simulink model "EVWITHOUTBOOSTCONVERTER"  (R2022a)
settings: Solver=ode23t  StartTime=0.0  StopTime=0.025  MaxStep=1e-3  RelTol=1e-3
undefined symbols (not defined in the file): Ion, Lithium
libraries: nesl_utility x14, fl_lib x12, sdl_lib x10, spsSeriesRLCBranchLib x5, spsDiodeLib x4, spsVoltageMeasurementLib x4, spsIGBTDiodeLib x4, simulink x3, spsMultimeterLib x3, spsPowerLib x2, spsACVoltageSourceLib x1, spsBatteryLib x1
settings Model: Creator=Arjun TM  LastModifiedBy=B SAI CHARAN TEJ
settings SolverCC: AlgebraicLoopSolver=TrustRegion
settings DataIOCC: ReturnWorkspaceOutputs=off
settings DebuggingCC: UnconnectedInputMsg=warning  UnconnectedOutputMsg=warning  UnconnectedLineMsg=warning  SFMachineParentedDataDiag=warning
settings RTWCC: DLArmComputeVersion=19.05

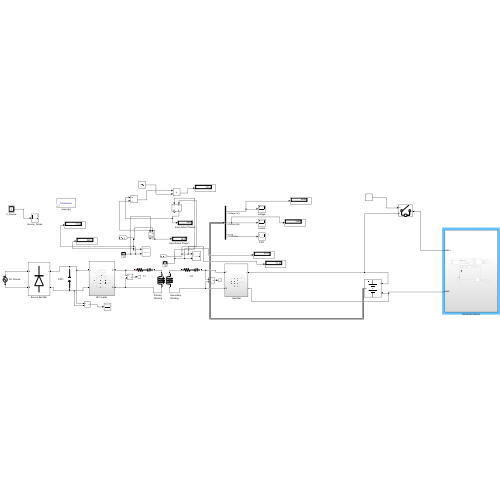
[thumbnail: Simulink's stored preview of the top-level diagram]
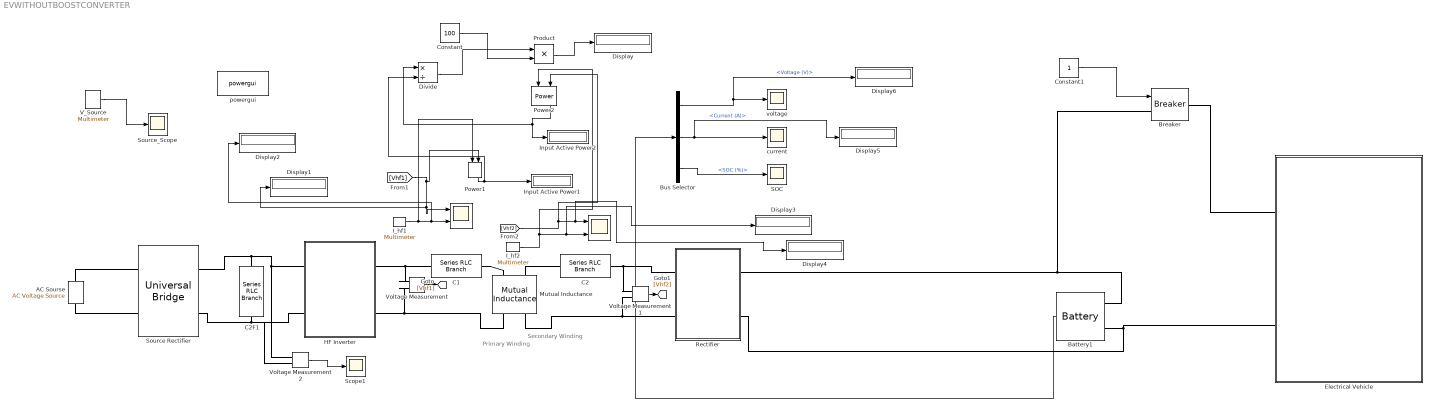
== system EVWITHOUTBOOSTCONVERTER ==
  note: Secondary
      | Winding
  note: Primary
      | Winding
  " " : Scope  NumInputPorts=2
  "   " : Scope  NumInputPorts=2
  " Rectifier" : Subsystem
  AC Sourse : spsACVoltageSourceLib/AC Voltage Source  Amplitude=230  Phase=0  Frequency=50  SampleTime=0  Measurements=Voltage  BusType=swing  Pref=10e3  Qref=0  Qmin=-inf  Qmax=+inf
  Battery1 : spsBatteryLib/Battery  BatType=Lithium-Ion  ShowTempParam=off  ThermalPreset=no  ShowAgeParam=off  NomV=72  NomQ=408.5  SOC=80  Batt_Tr=30  PresetModel=off  MaxQ=5.4  MinV=54  FullV=90.8071  Dis_rate=2.3478  R=0.13333  Normal_OP=4.8835  expZone="[85.7878     0.265304]"  current=[6.5 13 32.5]  Units=Time  Tci=20  NomT=20  T2=-30  MaxQ2=4.8  FullV2=7.1  Normal_OP2=5.655  expZone2="[6.58           1]"  Rca=0.6  ti=2000  Dp=0  Neq0=0  Tsim=1e6  Ta1=25  Qeol=5.4*0.9  Reol=0.013333*1.2  Char_age=[2.3478, 3]  Dis_age=[2.3478, 10]  N1=1500  N2=10500  N3=1000  N4=1400  Ta2=45  N5=950
  Breaker : spsBreakerLib/Breaker  InitialState=0  SwitchingTimes="[1/60  5/60]"  External=on  BreakerResistance=0.01  SnubberResistance=1e6  SnubberCapacitance=inf  Measurements=None  MoreParameters=on  NoBreakLoop=off
      settings: SourceProductBaseCode=PS
  Bus Selector : BusSelector  OutputSignals=Voltage (V),Current (A),SOC (%)
  C1 : spsSeriesRLCBranchLib/Series RLC Branch  LConnTagsString=__new0  RConnTagsString=__new0  BranchType=RC  Resistance=1e-6  Inductance=1e-3  SetiL0=off  InitialCurrent=0  Capacitance=105.74e-9  Setx0=off  InitialVoltage=0  Measurements=Branch current
  C2 : spsSeriesRLCBranchLib/Series RLC Branch  LConnTagsString=__new0  RConnTagsString=__new0  BranchType=RC  Resistance=0.001  Inductance=1e-3  SetiL0=off  InitialCurrent=0  Capacitance=109.69e-9  Setx0=off  InitialVoltage=0  Measurements=Branch current
  C2F1 : spsSeriesRLCBranchLib/Series RLC Branch  LConnTagsString=__new0  RConnTagsString=__new0  BranchType=C  Resistance=1e-6  Inductance=1e-3  SetiL0=off  InitialCurrent=0  Capacitance=500e-4  Setx0=off  InitialVoltage=0  Measurements=None
  Constant : Constant  Value=100
  Constant1 : Constant
  Display{,1..6} (7 alike) : Display
  Divide : Product  Inputs=*/
  Electrical Vehicle : Subsystem
  HF Inverter : Subsystem
  I_hf1 : spsMultimeterLib/Multimeter  L=15  sel=10  yselected={}  Gain=1  OutputType=Complex  PlotAtSimulationStop=off  PhasorSimulation=off
  I_hf2 : spsMultimeterLib/Multimeter  L=15  sel=11  yselected={}  Gain=1  OutputType=Complex  PlotAtSimulationStop=off  PhasorSimulation=off
  Input Active Power1 : Display
  Input Active Power2 : Display
  Mutual Inductance : spsMutualInductanceLib/Mutual Inductance  LConnTagsString=a|b  RConnTagsString=A|B  TypeOfMutual=Two or three windings with equal mutual terms  NumberOfWindings=3  SelfImpedance1=[1e-3 266.16e-6]  SelfImpedance2=[1e-3 256.79e-6]  ThreeWindings=off  SelfImpedance3=[ 1.1 1.1e-03]  MutualImpedance="[0  28.46e-6]"  InductanceMatrix="[1.0 0.9  0.9 ;  0.9 1.0  0.9;  0.9 0.9 1.0 ] * 1e-3"  ResistanceMatrix="[1.0 0.9  0.9 ;  0.9 1.0  0.9;  0.9 0.9 1.0 ]"  Measurements=None
      settings: SourceProductBaseCode=PS
  Power1 : spsPowerLib/Power  Freq=30000  Vinit=[1, 0]  Iinit=[1, 0]  Ts=0
      settings: SourceProductBaseCode=PS
  Power2 : spsPowerLib/Power  Freq=30000  Vinit=[1, 0]  Iinit=[1, 0]  Ts=0
      settings: SourceProductBaseCode=PS
  Product : Product
  SOC : Scope
  Scope1 : Scope
  Source Rectifier : spsUniversalBridgeLib/Universal Bridge  Arms=2  SnubberResistance=1e5  SnubberCapacitance=inf  Device=Diodes  Ron=1e-3  Lon=0  ForwardVoltages="[  0  0  ]"  ForwardVoltage=0  GTOparameters=[ 10e-6 , 20e-6 ]  IGBTparameters=[ 1e-6 , 2e-6 ]  Measurements=All voltages and currents  Measurements_2=None  converterType=Rectifier
  Source_Scope : Scope
  V_Source : spsMultimeterLib/Multimeter  L=15  sel=9  yselected={}  Gain=1  OutputType=Complex  PlotAtSimulationStop=off  PhasorSimulation=off
  Voltage Measurement : spsVoltageMeasurementLib/Voltage Measurement  PhasorSimulation=off  OutputType=Complex  PSBequivalent=0
  Voltage Measurement1 : spsVoltageMeasurementLib/Voltage Measurement  PhasorSimulation=off  OutputType=Complex  PSBequivalent=0
  Voltage Measurement2 : spsVoltageMeasurementLib/Voltage Measurement  PhasorSimulation=off  OutputType=Complex  PSBequivalent=0
  current : Scope
  powergui : spspowerguiLib/powergui  Priority=1  SimulationMode=Continuous  SampleTime=50e-5  frequency=60  Iterations=50  frequencyindice=0  Pbase=100e6  ErrMax=1e-4  UnitsV=kV  UnitsW=MW  buscounter=0  FunctionMessages=off  echomessages=off  EnableUseOfTLC=off  CurrentSourceSwitches=off  DisableSnubberDevices=off  DisableRonSwitches=off  DisableVfSwitches=off  DisplayEquations=off  AutomaticDiscreteSolvers=off  SolverType=Tustin/Backward Euler (TBE)  Interpol=off  ExternalGateDelay=off  methode=off  Ts=100  x0status=blocks  SPID=on  SwTol=0  HookPort=off  NonlinearTolerance=1e-4  nMaxIteration=100  ContinueOnMaxIteration=off  RestoreLinks=warning  ResistiveCurrentMeasurement=off  Frange=[0:2:500]  Ylog=off  Xlog=on  ShowGrid=off  save=off  variable=ZData  structure=source  ZoomFFT=off  StartTime=0.1  cycles=5  DisplayStyle=2  fundamental=50  FreqAxis=on  MaxFrequency=1000  frequencyindicesteady=1  RmsSteady=1  display=off
  voltage : Scope
  wires:
  V_Source/1 -> Source_Scope/1
  Voltage Measurement/1 -> [Vhf1]
  Voltage Measurement1/1 -> [Vhf2]
  I_hf2/1 -> Power2/2, Display3/1, "   "/2
  Bus Selector/3 -> SOC/1  "<SOC (%)>"
  Divide/1 -> Product/1
  Constant/1 -> Product/2
  Product/1 -> Display/1
  Voltage Measurement2/1 -> Scope1/1
  [Vhf1] -> Power1/1, Display1/1, " "/1
  I_hf1/1 -> Display2/1, " "/2, Power1/2
  Power1/1 -> Divide/2, Input Active Power1/1
  Battery1/1 -> Bus Selector/1
  Power2/1 -> Divide/1, Input Active Power2/1
  Bus Selector/2 -> Display5/1, current/1  "<Current (A)>"
  Constant1/1 -> Breaker/1
  [Vhf2] -> Power2/1, Display4/1, "   "/1
  Bus Selector/1 -> Display6/1, voltage/1  "<Voltage (V)>"
  connections:
  C1/RConn1 -- Mutual Inductance/LConn1
  Mutual Inductance/LConn2 -- C2/LConn1
  AC Sourse/LConn1 -- Source Rectifier/LConn2
  AC Sourse/RConn1 -- Source Rectifier/LConn1
  Source Rectifier/RConn2 -- Voltage Measurement2/LConn2 -- HF Inverter/LConn2 -- C2F1/RConn1
  C2F1/LConn1 -- Voltage Measurement2/LConn1 -- HF Inverter/LConn1 -- Source Rectifier/RConn1
  C1/LConn1 -- Voltage Measurement/LConn1 -- HF Inverter/RConn1
  Mutual Inductance/RConn1 -- Voltage Measurement/LConn2 -- HF Inverter/RConn2
  C2/RConn1 -- Voltage Measurement1/LConn1 -- " Rectifier"/LConn1
  Mutual Inductance/RConn2 -- Voltage Measurement1/LConn2 -- " Rectifier"/LConn2
  " Rectifier"/RConn2 -- Electrical Vehicle/LConn2 -- Battery1/LConn2
  Electrical Vehicle/LConn1 -- Breaker/RConn1
  " Rectifier"/RConn1 -- Breaker/LConn1 -- Battery1/LConn1

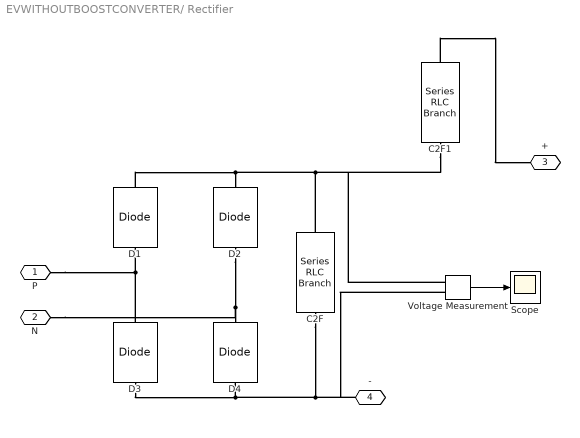
== system EVWITHOUTBOOSTCONVERTER/ Rectifier ==
  C2F : spsSeriesRLCBranchLib/Series RLC Branch  LConnTagsString=__new0  RConnTagsString=__new0  BranchType=C  Resistance=1e-6  Inductance=1e-3  SetiL0=off  InitialCurrent=0  Capacitance=300e-6  Setx0=off  InitialVoltage=0  Measurements=Branch voltage
  C2F1 : spsSeriesRLCBranchLib/Series RLC Branch  LConnTagsString=__new0  RConnTagsString=__new0  BranchType=R  Resistance=1e-6  Inductance=1e-3  SetiL0=off  InitialCurrent=0  Capacitance=300e-6  Setx0=off  InitialVoltage=0  Measurements=Branch voltage
  D{1..4} (4 alike) : spsDiodeLib/Diode  Ron=0.001  Lon=0  Vf=0.8  IC=0  UseSnubber=0  Rs=500  Cs=250e-9  Measurements=off
  Scope : Scope
  Voltage Measurement : spsVoltageMeasurementLib/Voltage Measurement  PhasorSimulation=off  OutputType=Complex  PSBequivalent=0
  P : PMIOPort  Side=Left
  N : PMIOPort  Port=2  Side=Left
  + : PMIOPort  Port=3  Side=Right
  - : PMIOPort  Port=4  Side=Right
  wires:
  Voltage Measurement/1 -> Scope/1
  connections:
  D1/RConn1 -- C2F1/RConn1 -- Voltage Measurement/LConn1 -- C2F/LConn1 -- D2/RConn1
  D3/RConn1 -- P/RConn1 -- D1/LConn1
  C2F/RConn1 -- Voltage Measurement/LConn2 -- -/RConn1 -- D3/LConn1 -- D4/LConn1
  D2/LConn1 -- N/RConn1 -- D4/RConn1
  C2F1/LConn1 -- +/RConn1

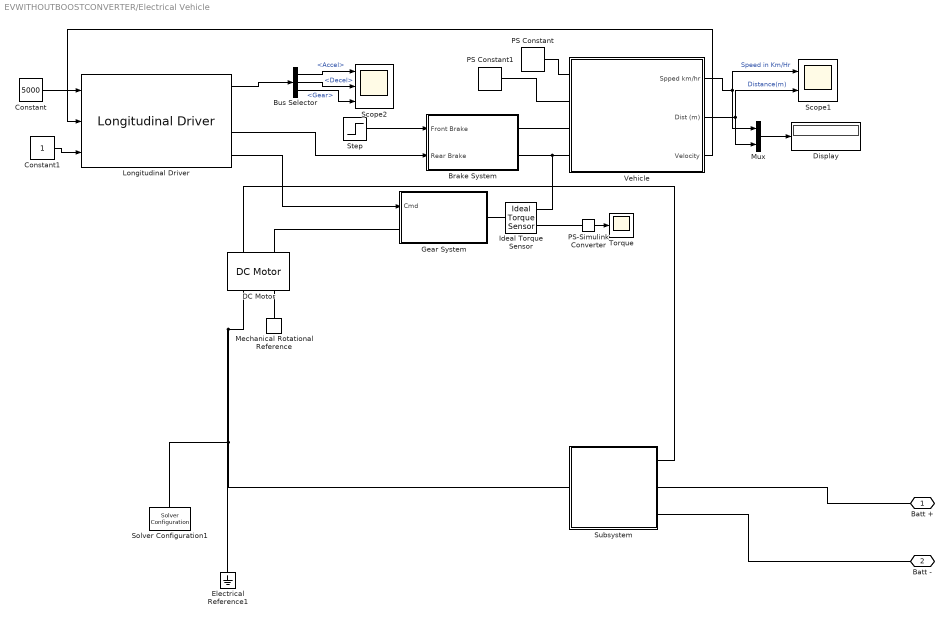
== system EVWITHOUTBOOSTCONVERTER/Electrical Vehicle ==
  Brake System : Subsystem
  Bus Selector : BusSelector  OutputSignals=Accel,Decel,Gear
  Constant : Constant  Value=5000
  Constant1 : Constant
  DC Motor : ee_lib/Electromechanical/Brushed Motors/DC Motor  field_option=ee.enum.field_option.pm  Rf=100 Ohm  Lf=1 H  Laf=0.15 H  If0=0 A  parameterization=ee.enum.dcparam_option.load_speed  Ra=3.9 Ohm  La=0.005 H  emf_or_torque=ee.enum.emf_or_torque.kv  Kv=0.072e-3 V/rpm  Ki=6.876e-4 N*m/A  T_stall=0.24e-3 N*m  w_max=9000 rpm  w_rated=8000 rpm  P_rated=5 kW  V_rated=72 V  lam_param=ee.enum.lam_param.damping  i_noload=0 A  V_i_noload=1.5 V  J=0.01 g*cm^2  lam=0 N*m/(rad/s)  speed0=0 rpm  enable_fault_armature=simscape.enum.onoff.off  rev_faulted=1 / 3  G_faulted_armature=1e-5 S  fault_trigger_armature=ee.enum.faults.faultTrigger.temporal  t_fault_armature=1 s  max_permissible_current_armature=inf A  t_fail_on_current_armature=1 s  enable_fault_field=simscape.enum.onoff.off  G_faulted_field=1e-5 S  fault_trigger_field=ee.enum.faults.faultTrigger.temporal  t_fault_field=1 s  max_permissible_current_field=inf A  t_fail_on_current_field=1 s  fault_action=simscape.enum.assert.action.none  alpha=3.93e-3 1/K  Tmeas=25 degC  thermal_mass=100 J/K  initial_temperature=25 degC
  Display : Display
  Electrical Reference1 : fl_lib/Electrical/Electrical Elements/Electrical Reference
  Gear System : Subsystem
  Ideal Torque Sensor : fl_lib/Mechanical/Mechanical Sensors/Ideal Torque Sensor
  Longitudinal Driver : autolibshared/Longitudinal Driver  extAccelOvr=off  extDecelOvr=off  extAccelHld=off  extDecelHld=off  extAccelZero=off  extDecelZero=off  cntrlType=PI  shftType=None  velUnits=m/s  gearOut=on  Kp=15  Ki=1  Kff=.05  Kg=.01  VehVelVec=[0 100]  KffVec=[.1 .1]  KpVec=[10 10]  KiVec=[5 5]  KgVec=[0 0]  m=1500  Kpt=3000  tau=.1  L=2  aR=200  bR=2.5  cR=.5  g=9.81  vnom=100  Kaw=.1  tauerr=.03  tauPt=2  GearInit=0  tShift=.1  pdlVec=[0.1 0.4 0.5 0.9]  upShftTbl=[-1 12.9375 26.4375 39.9375 51.18749999999999 62.4375 72.84375 83.25;-1 16.3125 29.8125 43.3125 54.5624 65.8125 76.78125 87.75;-1 19.6875 33.1875 46.68749999999999 57.9375 69.1875 80.71875 92.25;-1 33 52.5 77.25 100.5 138.75 161.875 185]  dwnShftTbl=[1 9.5625 23.0625 36.5625 47.8125 59.0625 68.90625 78.75;1 12.9375 26.4375 39.9375 51.18749999999999 62.4375 72.84375 83.25;1 16.3125 29.8125 43.3125 54.562499 65.8125 76.78125 87.75;1 19.6875 33.1875 46.68749999999999 57.9375 69.1875 80.71875 92.25]  tClutch=.5  tRev=.5  tPark=120  aMode=1  UpGearVec="[0  1  2  3  4  5  6  7]"  DownGearVec="[1  2  3  4  5  6  7  8]"
      settings: SourceProductBaseCode=PW,DR,MT,UV,VE
  Mechanical Rotational Reference : fl_lib/Mechanical/Rotational Elements/Mechanical Rotational Reference
  Mux : Mux  Inputs=2
  PS Constant : fl_lib/Physical Signals/Sources/PS Constant  constant=0
  PS Constant1 : fl_lib/Physical Signals/Sources/PS Constant  constant=0
  PS-Simulink Converter : nesl_utility/PS-Simulink Converter  PhysicalDomain=network_engine_domain  SubClassName=ps_output  LeftPortType=input  RightPortType=output  PseudoPeriodic=off  Frequencies=[]  VectorFormat=1-D array  Unit=inherit  AffineConversion=off
      settings: SourceProductBaseCode=PW,SS
  Scope1 : Scope  NumInputPorts=2
  Scope2 : Scope  NumInputPorts=3
  Solver Configuration1 : nesl_utility/Solver Configuration  PhysicalDomain=network_engine_domain  SubClassName=solver  LeftPortType=input  RightPortType=generic  Tones=[]  Harmonics=[]  SimulateNoise=off  Profile=off  UseLocalSampling=off  EnableSwitchedLinearOptims=on  FrequencyDomain=off  UseCCode=off  RelTol=0.001  AbsTol=1e-06  MinStep=1e-09  ToWorkspace=off  RevertToSquareIcSolve=off  NumHomotopyIterations=100  PhasorMode=off  PhasorModeNumHarmonics=1  IndexReductionMethod=DerivativeReplacement  DoDC=off  ResidualTolerance=1e-09  UseLocalSolver=off  LocalSolverChoice=NE_BACKWARD_EULER_ADVANCER  LocalSolverSampleTime=1e-7  DoFixedCost=on  MaxNonlinIter=3  MaxModeIter=2  ComputeImpulses=off  ImpulseIterations=2  LinearAlgebra=Sparse  LinearAlgebraNumThread=0  EquationFormulation=NE_TIME_EF  DelaysMemoryBudget=1024  AutomaticFiltering=on  FilteringTimeConstant=0.001  PartitionStorageMethod=AS_NEEDED  PartitionMemoryBudget=1024  PartitionMethod=FAST
      settings: SourceProductBaseCode=PW,SS
  Step : Step  Time=75  After=100  SampleTime=0
  Subsystem : Subsystem
  Torque : Scope
  Vehicle : Subsystem
  Batt + : PMIOPort  Side=Left
  Batt - : PMIOPort  Port=2  Side=Left
  wires:
  Step/1 -> Brake System/1(Front Brake)
  Bus Selector/2 -> Scope2/2  "<Decel>"
  Constant1/1 -> Longitudinal Driver/3
  Vehicle/2(Dist (m)) -> Mux/2, Scope1/2  "Distance(m)"
  PS-Simulink Converter/1 -> Torque/1
  Vehicle/1(Spped km/hr) -> Scope1/1, Mux/1  "Speed in Km/Hr"
  Bus Selector/1 -> Scope2/1  "<Accel>"
  Constant/1 -> Longitudinal Driver/1
  Longitudinal Driver/1 -> Bus Selector/1
  Mux/1 -> Display/1
  Vehicle/3(Velocity) -> Longitudinal Driver/2
  Longitudinal Driver/3 -> Brake System/2(Rear Brake)
  Longitudinal Driver/4 -> Gear System/1(Cmd)
  Bus Selector/3 -> Scope2/3  "<Gear>"
  connections:
  Solver Configuration1/RConn1 -- Electrical Reference1/LConn1 -- DC Motor/RConn1 -- Subsystem/LConn1
  PS Constant/RConn1 -- Vehicle/LConn1
  Brake System/RConn2 -- Ideal Torque Sensor/RConn1 -- Vehicle/LConn4
  PS Constant1/RConn1 -- Vehicle/LConn2
  Ideal Torque Sensor/RConn2 -- PS-Simulink Converter/LConn1
  Gear System/RConn1 -- Ideal Torque Sensor/LConn1
  Brake System/RConn1 -- Vehicle/LConn3
  Mechanical Rotational Reference/LConn1 -- DC Motor/RConn2
  Batt +/RConn1 -- Subsystem/RConn2
  Batt -/RConn1 -- Subsystem/RConn3
  Gear System/LConn1 -- DC Motor/LConn2
  DC Motor/LConn1 -- Subsystem/RConn1

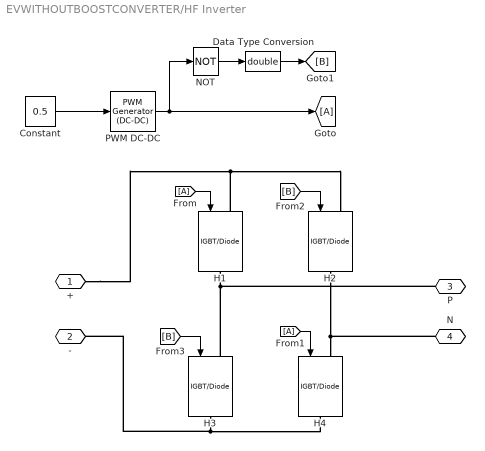
== system EVWITHOUTBOOSTCONVERTER/HF Inverter ==
  Constant : Constant  Value=0.5
  Data Type Conversion : DataTypeConversion  OutDataTypeStr=double  SaturateOnIntegerOverflow=off  RndMeth=Floor
  From : From
  From1 : From
  Goto : Goto
  H{1..4} (4 alike) : spsIGBTDiodeLib/IGBT//Diode  Ron=1e-3  Rs=1e5  Cs=inf  Measurements=off
  "NOT " : Logic  Operator=NOT  IconShape=distinctive  AllPortsSameDT=off  OutDataTypeStr=boolean
  PWM DC-DC : spsPWMGeneratorDCDCLib/PWM Generator (DC-DC)  Fsw=30000  Ts=0
  + : PMIOPort  Side=Left
  - : PMIOPort  Port=2  Side=Left
  P : PMIOPort  Port=3  Side=Right
  N : PMIOPort  Port=4  Side=Right
  wires:
  [B] -> H2/1
  [B] -> H3/1
  From1/1 -> H4/1
  From/1 -> H1/1
  "NOT "/1 -> Data Type Conversion/1
  Constant/1 -> PWM DC-DC/1
  Data Type Conversion/1 -> [B]
  PWM DC-DC/1 -> "NOT "/1, Goto/1
  connections:
  H1/LConn1 -- H2/LConn1 -- +/RConn1
  H2/RConn1 -- N/RConn1 -- H4/LConn1
  H3/RConn1 -- -/RConn1 -- H4/RConn1
  H3/LConn1 -- P/RConn1 -- H1/RConn1

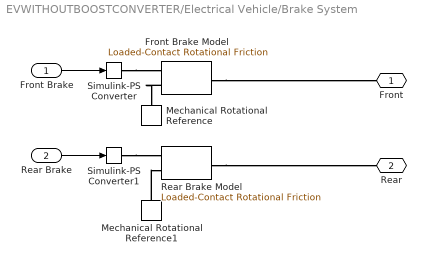
== system EVWITHOUTBOOSTCONVERTER/Electrical Vehicle/Brake System ==
  Front Brake : Inport
  Rear Brake : Inport  Port=2
  Front Brake Model : sdl_lib/Brakes & Detents/Rotational/Loaded-Contact Rotational Friction  geometry_model=sdl.enum.friction_geometry.radius  r_eff=280 mm  d_o=150 mm  d_i=100 mm  friction_model=sdl.enum.friction_model_TLU_thermal.fixed  mu_w_vector=[0, 100, 1000] rad/s  temperature_TLU=[280, 300, 320] K  mu_static=0.35  mu_static_vector=[.4, .38, .36]  mu_coulomb=0.3  mu_coulomb_vector=[.3, .22, .19]  mu_coulomb_temp_vector=[.3, .28, .25]  mu_coulomb_matrix=[.34, .32, .3; .3, .28, .25; .25, .2, .15]  mu_interp_method=simscape.enum.interpolation.linear  mu_extrap_method=simscape.enum.extrapolation.linear  w_tol=0.001 rad/s  force_min=1 N  mu_visc=0 N*m/(rad/s)  initial_state_locked=sdl.enum.initial_lock.unlocked  enable_faults=simscape.enum.onoff.off  fault_type=sdl.enum.clutchFault.lock  external_fault=simscape.enum.onoff.off  temporal_fault=simscape.enum.onoff.off  fault_time=5 s  report_fault=simscape.enum.assert.action.none  thermal_mass=50 kJ/K  T_init=300 K
      settings: SourceProductBaseCode=LD  InternalSimscapePortConfiguration="{\"Bottom\":[],\"Left\":[{\"id\":\"N\",\"label\":\"N\",\"type\":\"input\"},{\"id\":\"B\",\"label\":\"B\",\"type\":\"foundation.mechanical.rotational.rotational\"}],\"Right\":[{\"id\":\"F\",\"label\":\"F\",\"type\":\"foundation.mechanical.rotational.rotational\"}],\"Top\":[]}"
  Mechanical Rotational Reference : fl_lib/Mechanical/Rotational Elements/Mechanical Rotational Reference
  Mechanical Rotational Reference1 : fl_lib/Mechanical/Rotational Elements/Mechanical Rotational Reference
  Rear Brake Model : sdl_lib/Brakes & Detents/Rotational/Loaded-Contact Rotational Friction  geometry_model=sdl.enum.friction_geometry.radius  r_eff=280 mm  d_o=150 mm  d_i=100 mm  friction_model=sdl.enum.friction_model_TLU_thermal.fixed  mu_w_vector=[0, 100, 1000] rad/s  temperature_TLU=[280, 300, 320] K  mu_static=0.35  mu_static_vector=[.4, .38, .36]  mu_coulomb=0.3  mu_coulomb_vector=[.3, .22, .19]  mu_coulomb_temp_vector=[.3, .28, .25]  mu_coulomb_matrix=[.34, .32, .3; .3, .28, .25; .25, .2, .15]  mu_interp_method=simscape.enum.interpolation.linear  mu_extrap_method=simscape.enum.extrapolation.linear  w_tol=0.001 rad/s  force_min=1 N  mu_visc=0 N*m/(rad/s)  initial_state_locked=sdl.enum.initial_lock.unlocked  enable_faults=simscape.enum.onoff.off  fault_type=sdl.enum.clutchFault.lock  external_fault=simscape.enum.onoff.off  temporal_fault=simscape.enum.onoff.off  fault_time=5 s  report_fault=simscape.enum.assert.action.none  thermal_mass=50 kJ/K  T_init=300 K
      settings: SourceProductBaseCode=LD  InternalSimscapePortConfiguration="{\"Bottom\":[],\"Left\":[{\"id\":\"N\",\"label\":\"N\",\"type\":\"input\"},{\"id\":\"B\",\"label\":\"B\",\"type\":\"foundation.mechanical.rotational.rotational\"}],\"Right\":[{\"id\":\"F\",\"label\":\"F\",\"type\":\"foundation.mechanical.rotational.rotational\"}],\"Top\":[]}"
  Simulink-PS Converter : nesl_utility/Simulink-PS Converter  PhysicalDomain=network_engine_domain  SubClassName=ps_input  LeftPortType=input  RightPortType=output  PseudoPeriodic=off  Frequencies=[]  NoiseDistribution=none  NoiseParameters=[]  Unit=1  AffineConversion=off  FilteringAndDerivatives=provide  SimscapeFilterOrder=1  InputFilterTimeConstant=0.001  UdotUserProvided=0
      settings: SourceProductBaseCode=PW,SS
  Simulink-PS Converter1 : nesl_utility/Simulink-PS Converter  PhysicalDomain=network_engine_domain  SubClassName=ps_input  LeftPortType=input  RightPortType=output  PseudoPeriodic=off  Frequencies=[]  NoiseDistribution=none  NoiseParameters=[]  Unit=1  AffineConversion=off  FilteringAndDerivatives=provide  SimscapeFilterOrder=1  InputFilterTimeConstant=0.001  UdotUserProvided=0
      settings: SourceProductBaseCode=PW,SS
  Front : PMIOPort  Side=Right
  Rear : PMIOPort  Port=2  Side=Right
  wires:
  Rear Brake/1 -> Simulink-PS Converter1/1
  Front Brake/1 -> Simulink-PS Converter/1
  connections:
  Simulink-PS Converter1/RConn1 -- Rear Brake Model/LConn1
  Mechanical Rotational Reference1/LConn1 -- Rear Brake Model/LConn2
  Rear Brake Model/RConn1 -- Rear/RConn1
  Front Brake Model/LConn2 -- Mechanical Rotational Reference/LConn1
  Simulink-PS Converter/RConn1 -- Front Brake Model/LConn1
  Front Brake Model/RConn1 -- Front/RConn1

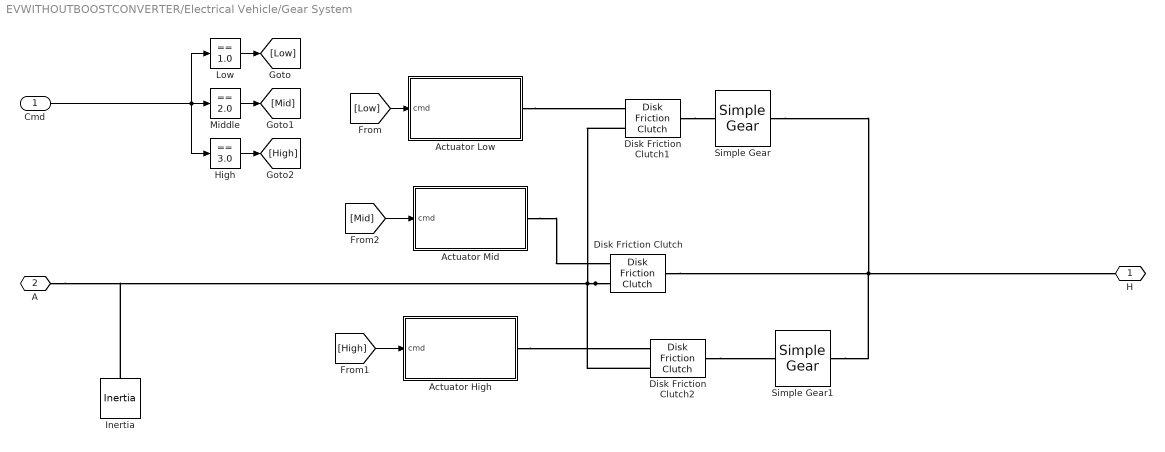
== system EVWITHOUTBOOSTCONVERTER/Electrical Vehicle/Gear System ==
  Cmd : Inport
  Actuator High : Subsystem
  Actuator Low : Subsystem
  Actuator Mid : Subsystem
  Disk Friction Clutch : sdl_lib/Clutches/Disk Friction Clutch  geometry_model=sdl.enum.friction_geometry.radius  r_eff=130 mm  d_o=150 mm  d_i=100 mm  nS=4  piston_area=0.001 m^2  unidirectional=sdl.enum.directionality.bidirectional  friction_model=sdl.enum.friction_model_TLU_thermal.fixed  mu_w_vector=[0, 100, 1000] rad/s  temperature_TLU=[280, 300, 320] K  mu_static=0.35  mu_static_vector=[.4, .38, .36]  mu_coulomb=0.3  mu_coulomb_vector=[.3, .22, .19]  mu_coulomb_temp_vector=[.3, .28, .25]  mu_coulomb_matrix=[.34, .32, .3; .3, .28, .25; .25, .2, .15]  mu_interp_method=simscape.enum.interpolation.linear  mu_extrap_method=simscape.enum.extrapolation.linear  d_f=1  w_tol=0.001 rad/s  pressure_min=100 Pa  mu_visc=0 N*m/(rad/s)  initial_state_locked=sdl.enum.initial_lock.unlocked  enable_faults=simscape.enum.onoff.off  fault_type=sdl.enum.clutchFault.lock  external_fault=simscape.enum.onoff.off  temporal_fault=simscape.enum.onoff.off  fault_time=5 s  report_fault=simscape.enum.assert.action.none  thermal_mass=50 kJ/K  T_init=300 K
      settings: SourceProductBaseCode=LD  InternalSimscapePortConfiguration="{\"Bottom\":[],\"Left\":[{\"id\":\"P\",\"label\":\"P\",\"type\":\"input\"},{\"id\":\"B\",\"label\":\"B\",\"type\":\"foundation.mechanical.rotational.rotational\"}],\"Right\":[{\"id\":\"F\",\"label\":\"F\",\"type\":\"foundation.mechanical.rotational.rotational\"}],\"Top\":[]}"
  Disk Friction Clutch1 : sdl_lib/Clutches/Disk Friction Clutch  geometry_model=sdl.enum.friction_geometry.radius  r_eff=130 mm  d_o=150 mm  d_i=100 mm  nS=4  piston_area=0.001 m^2  unidirectional=sdl.enum.directionality.bidirectional  friction_model=sdl.enum.friction_model_TLU_thermal.fixed  mu_w_vector=[0, 100, 1000] rad/s  temperature_TLU=[280, 300, 320] K  mu_static=0.35  mu_static_vector=[.4, .38, .36]  mu_coulomb=0.3  mu_coulomb_vector=[.3, .22, .19]  mu_coulomb_temp_vector=[.3, .28, .25]  mu_coulomb_matrix=[.34, .32, .3; .3, .28, .25; .25, .2, .15]  mu_interp_method=simscape.enum.interpolation.linear  mu_extrap_method=simscape.enum.extrapolation.linear  d_f=1  w_tol=0.001 rad/s  pressure_min=100 Pa  mu_visc=0 N*m/(rad/s)  initial_state_locked=sdl.enum.initial_lock.unlocked  enable_faults=simscape.enum.onoff.off  fault_type=sdl.enum.clutchFault.lock  external_fault=simscape.enum.onoff.off  temporal_fault=simscape.enum.onoff.off  fault_time=5 s  report_fault=simscape.enum.assert.action.none  thermal_mass=50 kJ/K  T_init=300 K
      settings: SourceProductBaseCode=LD  InternalSimscapePortConfiguration="{\"Bottom\":[],\"Left\":[{\"id\":\"P\",\"label\":\"P\",\"type\":\"input\"},{\"id\":\"B\",\"label\":\"B\",\"type\":\"foundation.mechanical.rotational.rotational\"}],\"Right\":[{\"id\":\"F\",\"label\":\"F\",\"type\":\"foundation.mechanical.rotational.rotational\"}],\"Top\":[]}"
  Disk Friction Clutch2 : sdl_lib/Clutches/Disk Friction Clutch  geometry_model=sdl.enum.friction_geometry.radius  r_eff=130 mm  d_o=150 mm  d_i=100 mm  nS=4  piston_area=0.001 m^2  unidirectional=sdl.enum.directionality.bidirectional  friction_model=sdl.enum.friction_model_TLU_thermal.fixed  mu_w_vector=[0, 100, 1000] rad/s  temperature_TLU=[280, 300, 320] K  mu_static=0.35  mu_static_vector=[.4, .38, .36]  mu_coulomb=0.3  mu_coulomb_vector=[.3, .22, .19]  mu_coulomb_temp_vector=[.3, .28, .25]  mu_coulomb_matrix=[.34, .32, .3; .3, .28, .25; .25, .2, .15]  mu_interp_method=simscape.enum.interpolation.linear  mu_extrap_method=simscape.enum.extrapolation.linear  d_f=1  w_tol=0.001 rad/s  pressure_min=100 Pa  mu_visc=0 N*m/(rad/s)  initial_state_locked=sdl.enum.initial_lock.unlocked  enable_faults=simscape.enum.onoff.off  fault_type=sdl.enum.clutchFault.lock  external_fault=simscape.enum.onoff.off  temporal_fault=simscape.enum.onoff.off  fault_time=5 s  report_fault=simscape.enum.assert.action.none  thermal_mass=50 kJ/K  T_init=300 K
      settings: SourceProductBaseCode=LD  InternalSimscapePortConfiguration="{\"Bottom\":[],\"Left\":[{\"id\":\"P\",\"label\":\"P\",\"type\":\"input\"},{\"id\":\"B\",\"label\":\"B\",\"type\":\"foundation.mechanical.rotational.rotational\"}],\"Right\":[{\"id\":\"F\",\"label\":\"F\",\"type\":\"foundation.mechanical.rotational.rotational\"}],\"Top\":[]}"
  High : simulink/Logic and Bit Operations/Compare To Constant  relop===  const=3.0  OutDataTypeStr=boolean
  Inertia : fl_lib/Mechanical/Rotational Elements/Inertia  inertia=0.01 kg*m^2  num_ports=foundation.enum.numPorts2.one  w_specify=off  w_priority=High  w=0 rad/s  w_nominal_specify=off  w_nominal_unit=rad/s  w_nominal_value=1  t_specify=off  t_priority=None  t=0 N*m  t_nominal_specify=off  t_nominal_unit=N*m  t_nominal_value=1
  Low : simulink/Logic and Bit Operations/Compare To Constant  relop===  const=1.0  OutDataTypeStr=boolean
  Middle : simulink/Logic and Bit Operations/Compare To Constant  relop===  const=2.0  OutDataTypeStr=boolean
  Simple Gear : sdl_lib/Gears/Simple Gear  ratio=3/2  rotation_direction=3-2*(1)  friction_model=sdl.enum.gear_efficiencies_load.off  T_noload=0.1 N*m  T_nom=5 N*m  efficiency_nom=0.8  efficiency=0.8  temperature_TLU=[280, 300, 320] K  load_TLU=[1, 5, 10] N*m  efficiency_TLU=[.95, .9, .85]  efficiency_TLU2=[.85, .8, .75; .95, .9, .85; .85, .8, .7]  w_thr=0.01 rad/s  pwr_thr=0.001 W  backlash_model=sdl.enum.backlashModel.Off  backlash_distance=1e-3 mm  x0=0 mm  r_base=0.1 m  hardstop_model=simscape.enum.hardstop.smooth  transition=1e-4 mm  backlash_stiffness=1e7 N/m  backlash_damping=1e6 N*s/m  e=0  v_tol=0.001 m/s  mu_visc=[0, 0] N*m/(rad/s)  enable_faults=simscape.enum.onoff.off  efficiency_fault=0.05  external_fault=simscape.enum.onoff.off  temporal_fault=simscape.enum.onoff.off  fault_time=5 s  fault_angles=pi / 12 rad  report_fault=(1)-1  thermal_mass=50 J/K  temperature_specify=off  temperature_priority=High  temperature=300 K  temperature_nominal_specify=off  temperature_nominal_unit=K  temperature_nominal_value=1  x_backlash_specify=off  x_backlash_priority=None  x_backlash=0 mm  x_backlash_nominal_specify=off  x_backlash_nominal_unit=mm  x_backlash_nominal_value=1  f_hardstop_specify=off  f_hardstop_priority=None  f_hardstop=0 N  f_hardstop_nominal_specify=off  f_hardstop_nominal_unit=N  f_hardstop_nominal_value=1  v_backlash_specify=off  v_backlash_priority=None  v_backlash=0 m/s  v_backlash_nominal_specify=off  v_backlash_nominal_unit=m/s  v_backlash_nominal_value=1
  Simple Gear1 : sdl_lib/Gears/Simple Gear  ratio=2/3  rotation_direction=3-2*(1)  friction_model=sdl.enum.gear_efficiencies_load.off  T_noload=0.1 N*m  T_nom=5 N*m  efficiency_nom=0.8  efficiency=0.8  temperature_TLU=[280, 300, 320] K  load_TLU=[1, 5, 10] N*m  efficiency_TLU=[.95, .9, .85]  efficiency_TLU2=[.85, .8, .75; .95, .9, .85; .85, .8, .7]  w_thr=0.01 rad/s  pwr_thr=0.001 W  backlash_model=sdl.enum.backlashModel.Off  backlash_distance=1e-3 mm  x0=0 mm  r_base=0.1 m  hardstop_model=simscape.enum.hardstop.smooth  transition=1e-4 mm  backlash_stiffness=1e7 N/m  backlash_damping=1e6 N*s/m  e=0  v_tol=0.001 m/s  mu_visc=[0, 0] N*m/(rad/s)  enable_faults=simscape.enum.onoff.off  efficiency_fault=0.05  external_fault=simscape.enum.onoff.off  temporal_fault=simscape.enum.onoff.off  fault_time=5 s  fault_angles=pi / 12 rad  report_fault=(1)-1  thermal_mass=50 J/K  temperature_specify=off  temperature_priority=High  temperature=300 K  temperature_nominal_specify=off  temperature_nominal_unit=K  temperature_nominal_value=1  x_backlash_specify=off  x_backlash_priority=None  x_backlash=0 mm  x_backlash_nominal_specify=off  x_backlash_nominal_unit=mm  x_backlash_nominal_value=1  f_hardstop_specify=off  f_hardstop_priority=None  f_hardstop=0 N  f_hardstop_nominal_specify=off  f_hardstop_nominal_unit=N  f_hardstop_nominal_value=1  v_backlash_specify=off  v_backlash_priority=None  v_backlash=0 m/s  v_backlash_nominal_specify=off  v_backlash_nominal_unit=m/s  v_backlash_nominal_value=1
  H : PMIOPort  Side=Right
  A : PMIOPort  Port=2  Side=Left
  wires:
  [High] -> Actuator High/1(cmd)
  Cmd/1 -> High/1, Middle/1, Low/1
  Middle/1 -> [Mid]
  Low/1 -> [Low]
  [Low] -> Actuator Low/1(cmd)
  High/1 -> [High]
  [Mid] -> Actuator Mid/1(cmd)
  connections:
  Actuator High/RConn1 -- Disk Friction Clutch2/LConn1
  Actuator Mid/RConn1 -- Disk Friction Clutch/LConn1
  Disk Friction Clutch/LConn2 -- Inertia/LConn1 -- A/RConn1 -- Disk Friction Clutch2/LConn2 -- Disk Friction Clutch1/LConn2
  Actuator Low/RConn1 -- Disk Friction Clutch1/LConn1
  Disk Friction Clutch/RConn1 -- H/RConn1 -- Simple Gear/RConn1 -- Simple Gear1/RConn1
  Disk Friction Clutch1/RConn1 -- Simple Gear/LConn1
  Disk Friction Clutch2/RConn1 -- Simple Gear1/LConn1

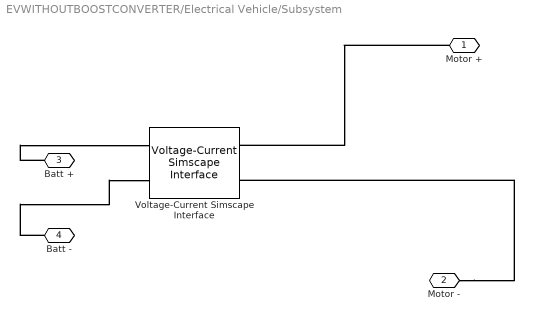
== system EVWITHOUTBOOSTCONVERTER/Electrical Vehicle/Subsystem ==
  Voltage-Current Simscape Interface : spsVoltageCurrentSimscapeInterfaceLib/Voltage-Current Simscape Interface  DFT=off  Fmode=First-order input filtering  T=1e-6  Ts=50e-6  i0=0  v0=0  Sd=Specialized Power Systems side  Measurements=off
      settings: SourceProductBaseCode=PS
  Motor + : PMIOPort  Side=Right
  Motor - : PMIOPort  Port=2  Side=Left
  Batt + : PMIOPort  Port=3  Side=Right
  Batt - : PMIOPort  Port=4  Side=Right
  connections:
  Motor -/RConn1 -- Voltage-Current Simscape Interface/RConn2
  Batt +/RConn1 -- Voltage-Current Simscape Interface/LConn1
  Batt -/RConn1 -- Voltage-Current Simscape Interface/LConn2
  Motor +/RConn1 -- Voltage-Current Simscape Interface/RConn1

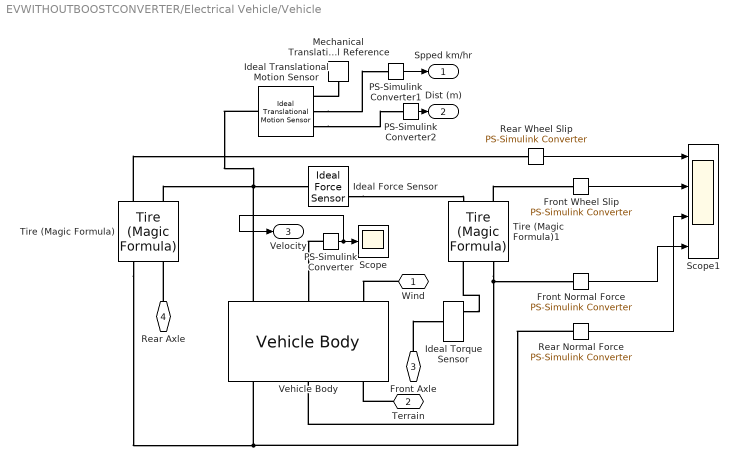
== system EVWITHOUTBOOSTCONVERTER/Electrical Vehicle/Vehicle ==
  Front Normal Force : nesl_utility/PS-Simulink Converter  PhysicalDomain=network_engine_domain  SubClassName=ps_output  LeftPortType=input  RightPortType=output  PseudoPeriodic=off  Frequencies=[]  VectorFormat=1-D array  Unit=N  AffineConversion=off
      settings: SourceProductBaseCode=PW,SS
  Front Wheel Slip : nesl_utility/PS-Simulink Converter  PhysicalDomain=network_engine_domain  SubClassName=ps_output  LeftPortType=input  RightPortType=output  PseudoPeriodic=off  Frequencies=[]  VectorFormat=1-D array  Unit=m  AffineConversion=off
      settings: SourceProductBaseCode=PW,SS
  Ideal Force Sensor : fl_lib/Mechanical/Mechanical Sensors/Ideal Force Sensor
  Ideal Torque Sensor : fl_lib/Mechanical/Mechanical Sensors/Ideal Torque Sensor
  Ideal Translational Motion Sensor : fl_lib/Mechanical/Mechanical Sensors/Ideal Translational Motion Sensor  offset=0 m
  Mechanical Translational Reference : fl_lib/Mechanical/Translational Elements/Mechanical Translational Reference
  PS-Simulink Converter : nesl_utility/PS-Simulink Converter  PhysicalDomain=network_engine_domain  SubClassName=ps_output  LeftPortType=input  RightPortType=output  PseudoPeriodic=off  Frequencies=[]  VectorFormat=1-D array  Unit=inherit  AffineConversion=off
      settings: SourceProductBaseCode=PW,SS
  PS-Simulink Converter1 : nesl_utility/PS-Simulink Converter  PhysicalDomain=network_engine_domain  SubClassName=ps_output  LeftPortType=input  RightPortType=output  PseudoPeriodic=off  Frequencies=[]  VectorFormat=1-D array  Unit=km/hr  AffineConversion=off
      settings: SourceProductBaseCode=PW,SS
  PS-Simulink Converter2 : nesl_utility/PS-Simulink Converter  PhysicalDomain=network_engine_domain  SubClassName=ps_output  LeftPortType=input  RightPortType=output  PseudoPeriodic=off  Frequencies=[]  VectorFormat=1-D array  Unit=m  AffineConversion=off
      settings: SourceProductBaseCode=PW,SS
  Rear Normal Force : nesl_utility/PS-Simulink Converter  PhysicalDomain=network_engine_domain  SubClassName=ps_output  LeftPortType=input  RightPortType=output  PseudoPeriodic=off  Frequencies=[]  VectorFormat=1-D array  Unit=N  AffineConversion=off
      settings: SourceProductBaseCode=PW,SS
  Rear Wheel Slip : nesl_utility/PS-Simulink Converter  PhysicalDomain=network_engine_domain  SubClassName=ps_output  LeftPortType=input  RightPortType=output  PseudoPeriodic=off  Frequencies=[]  VectorFormat=1-D array  Unit=N  AffineConversion=off
      settings: SourceProductBaseCode=PW,SS
  Scope : Scope
  Scope1 : Scope  NumInputPorts=4
  Tire (Magic Formula) : sdl_lib/Tires & Vehicles/Tire (Magic Formula)  parameterization=sdl.enum.magic_tire_model.constant  F_z1=3000 N  F_x1=3500 N  kappa1=10  B_m=10  C_m=1.9  D_m=1  E_m=0.97  fz0=4000 N  p_Cx=1.685  p_Dx=[1.21, -.037]  p_Ex=[.344, .095, -.02, 0]  p_Kx=[21.51, -.163, .245]  p_Hx=[-.002, .002]  p_Vx=[0, 0]  r_e=9 in  model_compliance=0  stiffness=1e6 N/m  damping=1000 N/(m/s)  model_inertia=1  inertia=1e-3 kg*m^2  initial_velocity=500 rad/s  model_resistance=1  resistance_model=1  coeff=0.005  p_tire=250e3 Pa  alpha=-0.003  beta=0.97  coeff_a=84e-4  coeff_b=6.2e-4 s/m  coeff_c=1.6e-4 s^2/m^2  v_thr=0.001 m/s  v_tr_thr=0.1 m/s
  Tire (Magic Formula)1 : sdl_lib/Tires & Vehicles/Tire (Magic Formula)  parameterization=sdl.enum.magic_tire_model.constant  F_z1=3000 N  F_x1=3500 N  kappa1=10  B_m=10  C_m=1.9  D_m=1  E_m=0.97  fz0=4000 N  p_Cx=1.685  p_Dx=[1.21, -.037]  p_Ex=[.344, .095, -.02, 0]  p_Kx=[21.51, -.163, .245]  p_Hx=[-.002, .002]  p_Vx=[0, 0]  r_e=9 in  model_compliance=0  stiffness=1e6 N/m  damping=1000 N/(m/s)  model_inertia=1  inertia=1e-3 kg*m^2  initial_velocity=500 rad/s  model_resistance=1  resistance_model=1  coeff=0.005  p_tire=250e3 Pa  alpha=-0.003  beta=0.97  coeff_a=84e-4  coeff_b=6.2e-4 s/m  coeff_c=1.6e-4 s^2/m^2  v_thr=0.001 m/s  v_tr_thr=0.1 m/s
  Vehicle Body : sdl_lib/Tires & Vehicles/Vehicle Body  mass=80+237 kg  n_w=1  x_f=1520 mm  x_r=1400 mm  y_c=254 mm  mass_var=simscape.enum.onoff.off  g=9.81 m/s^2  liftoff_warning=simscape.enum.onoff.off  area=1.33 m^2  Cd=1.2  rho=1.18 kg/m^3  model_pitch=simscape.enum.onoff.off  inertia=4000 kg*m^2  suspension_model=sdl.enum.linearTLU.linear  k_f=1e4 N/m  b_f=1e4 N/(m/s)  k_r=1e4 N/m  b_r=1e4 N/(m/s)  k_f_TLU=[-2000, -1000, 0, 1000, 2000] N  x_f_TLU=[-.4, -.2, 0, .2, .4] m  b_f_TLU=[-200, -100, 0, 100, 200] N  v_f_TLU=[-4, -2, 0, 2, 4] m/s  k_r_TLU=[-2000, -1000, 0, 1000, 2000] N  x_r_TLU=[-.4, -.2, 0, .2, .4] m  b_r_TLU=[-200, -100, 0, 100, 200] N  v_r_TLU=[-4, -2, 0, 2, 4] m/s  interp_method=simscape.enum.interpolation.linear  extrap_method=simscape.enum.extrapolation.linear  model_hardstop=simscape.enum.onoff.off  upper_bound_f=.25 m  lower_bound_f=-.25 m  stop_k_f=1e6 N/m  stop_b_f=150 N/(m/s)  upper_bound_r=.25 m  lower_bound_r=-.25 m  stop_k_r=1e6 N/m  stop_b_r=150 N/(m/s)  initial_pitch=0 rad  initial_pitch_rate=0 rad/s  v_specify=off  v_priority=High  v=0 m/s  v_nominal_specify=off  v_nominal_unit=m/s  v_nominal_value=1
  Wind : PMIOPort  Side=Left
  "Terrain " : PMIOPort  Port=2  Side=Left
  Front Axle : PMIOPort  Port=3  Side=Left
  Rear Axle : PMIOPort  Port=4  Side=Left
  Spped km/hr : Outport
  Dist (m) : Outport  Port=2
  Velocity : Outport  Port=3
  wires:
  PS-Simulink Converter1/1 -> Spped km/hr/1
  PS-Simulink Converter/1 -> Velocity/1, Scope/1
  PS-Simulink Converter2/1 -> Dist (m)/1
  Rear Wheel Slip/1 -> Scope1/1
  Front Wheel Slip/1 -> Scope1/2
  Rear Normal Force/1 -> Scope1/3
  Front Normal Force/1 -> Scope1/4
  connections:
  Rear Axle/RConn1 -- Tire (Magic Formula)/LConn2
  Tire (Magic Formula)/LConn1 -- Vehicle Body/RConn1 -- Rear Normal Force/LConn1
  Mechanical Translational Reference/LConn1 -- Ideal Translational Motion Sensor/RConn1
  Vehicle Body/LConn1 -- Ideal Translational Motion Sensor/LConn1 -- Ideal Force Sensor/LConn1 -- Tire (Magic Formula)/RConn2
  Tire (Magic Formula)1/LConn1 -- Vehicle Body/RConn2 -- Front Normal Force/LConn1
  Ideal Translational Motion Sensor/RConn3 -- PS-Simulink Converter2/LConn1
  PS-Simulink Converter/LConn1 -- Vehicle Body/LConn2
  Ideal Translational Motion Sensor/RConn2 -- PS-Simulink Converter1/LConn1
  Wind/RConn1 -- Vehicle Body/LConn3
  "Terrain "/RConn1 -- Vehicle Body/RConn3
  Front Axle/RConn1 -- Ideal Torque Sensor/LConn1
  Ideal Torque Sensor/RConn1 -- Tire (Magic Formula)1/LConn2
  Tire (Magic Formula)1/RConn1 -- Front Wheel Slip/LConn1
  Ideal Force Sensor/RConn1 -- Tire (Magic Formula)1/RConn2
  Tire (Magic Formula)/RConn1 -- Rear Wheel Slip/LConn1

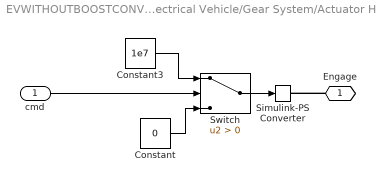
== system EVWITHOUTBOOSTCONVERTER/Electrical Vehicle/Gear System/Actuator High ==
  cmd : Inport
  Constant : Constant  Value=0
  Constant3 : Constant  Value=1e7
  Simulink-PS Converter : nesl_utility/Simulink-PS Converter  PhysicalDomain=network_engine_domain  SubClassName=ps_input  LeftPortType=input  RightPortType=output  PseudoPeriodic=off  Frequencies=[]  NoiseDistribution=none  NoiseParameters=[]  Unit=1  AffineConversion=off  FilteringAndDerivatives=provide  SimscapeFilterOrder=1  InputFilterTimeConstant=0.001  UdotUserProvided=0
      settings: SourceProductBaseCode=PW,SS
  Switch : Switch  Criteria=u2 > Threshold  SaturateOnIntegerOverflow=off  InputSameDT=off
  Engage : PMIOPort  Side=Right
  wires:
  Constant/1 -> Switch/3
  cmd/1 -> Switch/2
  Constant3/1 -> Switch/1
  Switch/1 -> Simulink-PS Converter/1
  connections:
  Engage/RConn1 -- Simulink-PS Converter/RConn1

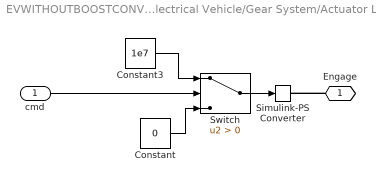
== system EVWITHOUTBOOSTCONVERTER/Electrical Vehicle/Gear System/Actuator Low ==
  cmd : Inport
  Constant : Constant  Value=0
  Constant3 : Constant  Value=1e7
  Simulink-PS Converter : nesl_utility/Simulink-PS Converter  PhysicalDomain=network_engine_domain  SubClassName=ps_input  LeftPortType=input  RightPortType=output  PseudoPeriodic=off  Frequencies=[]  NoiseDistribution=none  NoiseParameters=[]  Unit=1  AffineConversion=off  FilteringAndDerivatives=provide  SimscapeFilterOrder=1  InputFilterTimeConstant=0.001  UdotUserProvided=0
      settings: SourceProductBaseCode=PW,SS
  Switch : Switch  Criteria=u2 > Threshold  SaturateOnIntegerOverflow=off  InputSameDT=off
  Engage : PMIOPort  Side=Right
  wires:
  Constant/1 -> Switch/3
  cmd/1 -> Switch/2
  Constant3/1 -> Switch/1
  Switch/1 -> Simulink-PS Converter/1
  connections:
  Engage/RConn1 -- Simulink-PS Converter/RConn1

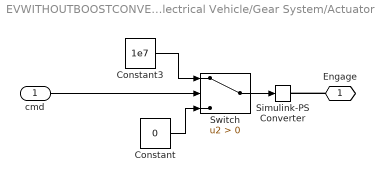
== system EVWITHOUTBOOSTCONVERTER/Electrical Vehicle/Gear System/Actuator Mid ==
  cmd : Inport
  Constant : Constant  Value=0
  Constant3 : Constant  Value=1e7
  Simulink-PS Converter : nesl_utility/Simulink-PS Converter  PhysicalDomain=network_engine_domain  SubClassName=ps_input  LeftPortType=input  RightPortType=output  PseudoPeriodic=off  Frequencies=[]  NoiseDistribution=none  NoiseParameters=[]  Unit=1  AffineConversion=off  FilteringAndDerivatives=provide  SimscapeFilterOrder=1  InputFilterTimeConstant=0.001  UdotUserProvided=0
      settings: SourceProductBaseCode=PW,SS
  Switch : Switch  Criteria=u2 > Threshold  SaturateOnIntegerOverflow=off  InputSameDT=off
  Engage : PMIOPort  Side=Right
  wires:
  Switch/1 -> Simulink-PS Converter/1
  Constant3/1 -> Switch/1
  cmd/1 -> Switch/2
  Constant/1 -> Switch/3
  connections:
  Engage/RConn1 -- Simulink-PS Converter/RConn1
